simulink model "DC_Motor"  (R2024b)
settings: Solver=VariableStepAuto  StartTime=0.0  StopTime=10.0  RelTol=1e-3
values from neighbouring files (symbols this model uses):
  b = 3.5077E-6    (= 3.5077e-06)    [DC_Motor_run.m]    (also in PID_Controlled_SPD_run.m = 10; run_SMD_Laplace.m = 0.1; run_Spring_mass_Damper.m = 10)
  J = 3.2284E-6    (= 3.2284e-06)    [DC_Motor_run.m]
  Kb = 0.0274    [DC_Motor_run.m]
  Kd = -7.6037e-04    (= -0.00076037)    [DC_Motor_run.m]    (also in PID_Controlled_SPD_run.m = 0; run_Spring_mass_Damper.m = 50)
  Ki = 0.0539    [DC_Motor_run.m]    (also in PID_Controlled_SPD_run.m = 0; run_Spring_mass_Damper.m = 300)
  Kp = 0.0247    [DC_Motor_run.m]    (also in PID_Controlled_SPD_run.m = 2000; run_Spring_mass_Damper.m = 350)
  Kt = 0.0274    [DC_Motor_run.m]
  L = 2.75E-6    (= 2.75e-06)    [DC_Motor_run.m]
  R = 4    [DC_Motor_run.m]
libraries: slpidlib x1
settings Model: Creator=sajim  LastModifiedBy=sajim

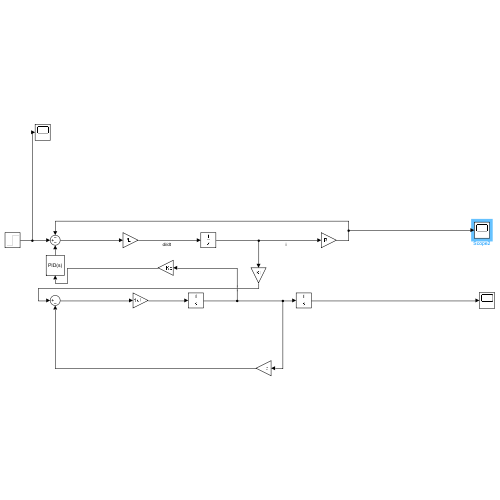
[thumbnail: Simulink's stored preview of the top-level diagram]
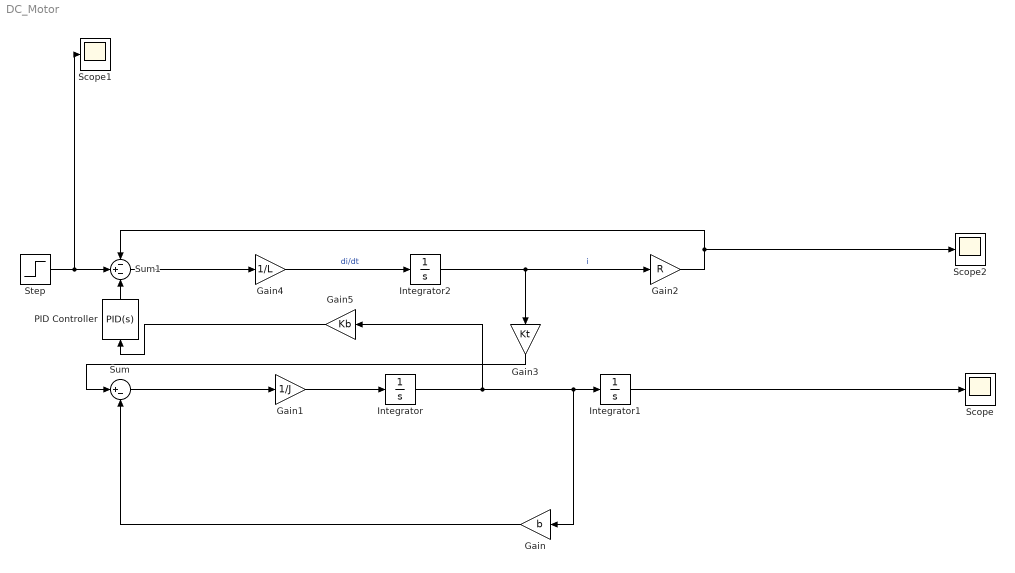
== system DC_Motor ==
  Gain : Gain  Gain=b
  Gain1 : Gain  Gain=1/J
  Gain2 : Gain  Gain=R
  Gain3 : Gain  Gain=Kt
  Gain4 : Gain  Gain=1/L
  Gain5 : Gain  Gain=Kb
  Integrator : Integrator
  Integrator1 : Integrator
  Integrator2 : Integrator
  PID Controller : slpidlib/PID Controller  Controller=PID  Form=Parallel  TimeDomain=Continuous-time  UseExternalTs=off  SampleTime=-1  IntegratorMethod=Forward Euler  FilterMethod=Forward Euler  ControllerParametersSource=internal  P=Kp  I=Ki  UseKiTs=off  D=Kd  UseExternalDerivativeSource=off  N=3.2951613909972  UseFilter=on  TunerSelectOption=Transfer Function Based (PID Tuner App)  InitialConditionSource=internal  InitialConditionForIntegrator=0  InitialConditionForFilter=0  DifferentiatorICPrevScaledInput=0  ExternalReset=none  TrackingMode=off  Kt=1  LimitOutput=off  SatLimitsSource=internal  UpperSaturationLimit=inf  LowerSaturationLimit=-inf  LinearizeAsGain=on  AntiWindupMode=none  Kb=1  LimitIntegrator=off  UpperIntegratorSaturationLimit=inf  LowerIntegratorSaturationLimit=-inf  POutMin=[]  POutMax=[]  IOutMin=[]  IOutMax=[]  DOutMin=[]  DOutMax=[]  NOutMin=[]  NOutMax=[]  SumOutMin=[]  SumOutMax=[]  SaturationOutMin=[]  SaturationOutMax=[]  PParamMin=[]  PParamMax=[]  IParamMin=[]  IParamMax=[]  DParamMin=[]  DParamMax=[]  NParamMin=[]  NParamMax=[]  KbParamMin=[]  KbParamMax=[]  KtParamMin=[]  KtParamMax=[]  KbOutMin=[]  KbOutMax=[]  KtOutMin=[]  KtOutMax=[]  IntegratorOutMin=[]  IntegratorOutMax=[]  FilterOutMin=[]  FilterOutMax=[]  SumI1OutMin=[]  SumI1OutMax=[]  SumI2OutMin=[]  SumI2OutMax=[]  SumI3OutMin=[]  SumI3OutMax=[]  SumI4OutMin=[]  SumI4OutMax=[]  SumDOutMin=[]  SumDOutMax=[]  DifferentiatorOutMin=[]  DifferentiatorOutMax=[]  FilterDiffOutCoefMin=[]  FilterDiffOutCoefMax=[]  ReciprocalOutMin=[]  ReciprocalOutMax=[]  SumDenOutMin=[]  SumDenOutMax=[]  SumNumOutMin=[]  SumNumOutMax=[]  DivideOutMin=[]  DivideOutMax=[]  UdiffTsProdOutMin=[]  UdiffTsProdOutMax=[]  NTsProdOutMin=[]  NTsProdOutMax=[]  UintegralTsProdOutMin=[]  UintegralTsProdOutMax=[]  UngainTsProdOutMin=[]  UngainTsProdOutMax=[]  ClampingZeroOutDataTypeStr=Inherit: Inherit via back propagation  ClampingZeroOutMin=[]  ClampingZeroOutMax=[]  FilterDenConstantOutDataTypeStr=Inherit: Inherit via back propagation  FilterDenConstantOutMin=[]  FilterDenConstantOutMax=[]  PCopyOutDataTypeStr=Inherit: Inherit via back propagation  PCopyOutMin=[]  PCopyOutMax=[]  NCopyOutDataTypeStr=Inherit: Inherit via back propagation  NCopyOutMin=[]  NCopyOutMax=[]  IntegratorContinuousStateAttributes=''  IntegratorStateMustResolveToSignalObject=off  IntegratorRTWStateStorageClass=Auto  FilterContinuousStateAttributes=''  FilterStateMustResolveToSignalObject=off  FilterRTWStateStorageClass=Auto  ParallelPVariant=InternalParameters  IdealPVariant=Disabled  IVariant=InternalParameters  DVariant=InternalParameters  IntegratorVariant=Continuous  SatVariant=Disabled  AWVariant=Passthrough  PCopyVariant=Disabled  TRVariant=Disabled  FdbkBlocksVariant=Forward  IdealPFdbkVariant=Disabled  SatFdbkVariant=Disabled  DerivativeFilterVariant=ContFilter  NVariant=InternalParameters  NCopyVariant=Disabled  FilterICVariant=InternalICsFilter  IntegratorICVariant=InternalICs  ExternalResetVariant=Disabled  TRSumVariant=Passthrough  SumFdbkVariant=Disabled  SumVariant=Sum_PID  TsampFilterVariant=InternalTs  TsampNgainVariant=Passthrough  TsampIntegralVariant=Disabled_SignalSpec  ExternalSaturationOutDataTypeStr=Inherit: Same as second input  DerivativeSourceVariant=ErrorSignal  PreIntVariant=InternalPreInt
  Scope : Scope
  Scope1 : Scope
  Scope2 : Scope
  Step : Step  SampleTime=0
  Sum : Sum  Inputs=|+-
  Sum1 : Sum  Inputs=-+-
  wires:
  Integrator/1 -> Gain5/1, Gain/1, Integrator1/1
  Integrator1/1 -> Scope/1
  Gain1/1 -> Integrator/1
  Gain/1 -> Sum/2
  Gain4/1 -> Integrator2/1  "di/dt"
  Integrator2/1 -> Gain3/1, Gain2/1  "i"
  Gain3/1 -> Sum/1
  Gain2/1 -> Scope2/1, Sum1/1
  Step/1 -> Scope1/1, Sum1/2
  Gain5/1 -> PID Controller/1
  Sum/1 -> Gain1/1
  Sum1/1 -> Gain4/1
  PID Controller/1 -> Sum1/3
